simulink model "PBVS_SoftHand"  (R2020b)
settings: Solver=VariableStepAuto  StartTime=0.0  StopTime=10  RelTol=1e-3
model workspace (MAT data in the model file):
  SL_ROS_VariableLengthArrays_MaxSizes.CommonInfo.ArrayTruncateAction = 'EmitWarning'
  SL_ROS_VariableLengthArrays_MaxSizes.MsgTypeMap = containers.Map
  SL_ROS_VariableLengthArrays_MaxSizes.MsgTypeMap.serialization.keys = {'sensor_msgs/Image'}
  SL_ROS_VariableLengthArrays_MaxSizes.MsgTypeMap.serialization.values{1}(1).PropertyName = 'Data'
  SL_ROS_VariableLengthArrays_MaxSizes.MsgTypeMap.serialization.values{1}(1).DataType = 'uint8'
  SL_ROS_VariableLengthArrays_MaxSizes.MsgTypeMap.serialization.values{1}(1).MaxLength = 2800000
  SL_ROS_VariableLengthArrays_MaxSizes.MsgTypeMap.serialization.values{1}(2).PropertyName = 'Encoding'
  SL_ROS_VariableLengthArrays_MaxSizes.MsgTypeMap.serialization.values{1}(2).DataType = 'uint8'
  SL_ROS_VariableLengthArrays_MaxSizes.MsgTypeMap.serialization.values{1}(2).MaxLength = 128
  SL_ROS_VariableLengthArrays_MaxSizes.MsgTypeMap.serialization.uniformity = 0
  SL_ROS_VariableLengthArrays_MaxSizes.MsgTypeMap.serialization.keyType = 'char'
  SL_ROS_VariableLengthArrays_MaxSizes.MsgTypeMap.serialization.valueType = 'any'
values from neighbouring files (symbols this model uses):
  camera_offset = rot(pi, 0, 0) * [-0.10; 0.0; -0.10]    [init_PBVS_SoftHand.m]
  dT = 1/frequency    (= 0.01)    [init_PBVS_SoftHand.m]
  DT = 1/20    (= 0.05)    [init_PBVS_SoftHand.m]
  f = 0.0019    [init_PBVS_SoftHand.m]
  init_pose = [position(1:3); orientation']    [init_PBVS_SoftHand.m]
  Kd = 0.*eye(6)    [init_PBVS_SoftHand.m]
  Kh = eye(7)    [init_PBVS_SoftHand.m]
  Kp = 1.0*eye(6)    [init_PBVS_SoftHand.m]
  l1 = 0.06    [init_PBVS_SoftHand.m]
  l2 = 0.04    [init_PBVS_SoftHand.m]
  O = [0; 0; 0]    [init_PBVS_SoftHand.m]
  o = [0; 0; pi/2-pi/8]    [init_PBVS_SoftHand.m]
  p = [0.5; 0.4; 0.1]    [init_PBVS_SoftHand.m]
  P0 = eye(6)*1    [init_PBVS_SoftHand.m]
  plane_x = 0.008    [init_PBVS_SoftHand.m]
  plane_y = 0.004    [init_PBVS_SoftHand.m]
  Q = zeros(6)    [init_PBVS_SoftHand.m]
  q_init = [ (0.0) (-pi/8) (0.0) (-pi/2-pi/6) (0.0) (pi/2+pi/24) (0.0) ]    [init_PBVS_SoftHand.m]
  R = eye(6)*0.0001    [init_PBVS_SoftHand.m]
  R_cam = rot(phi, theta, psi)    [init_PBVS_SoftHand.m]
  ref = [0; 0; 0.1; 0;  0; -pi]    [init_PBVS_SoftHand.m]
  st = 0.05    [init_PBVS_SoftHand.m]
libraries: simulink x2, robotmaniplib x2
settings Model: Creator=Acer  LastModifiedBy=Acer
settings OptimizationCC: EnhancedBackFolding=on  PassReuseOutputArgsAs=Individual arguments  ZeroExternalMemoryAtStartup=off  ZeroInternalMemoryAtStartup=off  MaxStackSize=64  OptimizeBlockOrder=speed  DifferentSizesBufferReuse=on  OptimizationCustomize=off  EfficientTunableParamExpr=on
settings DebuggingCC: ParameterTunabilityLossMsg=error
settings HardwareCC: ProdBitPerPointer=32  ProdBitPerSizeT=32  ProdBitPerPtrDiffT=32  ProdLargestAtomicFloat=None  ProdIntDivRoundTo=Undefined  ProdEndianess=Unspecified  ProdWordSize=32  ProdHWDeviceType=Generic->Unspecified (assume 32-bit Generic)  UseEmbeddedCoderFeatures=off
settings SFSimCC: MATLABDynamicMemAlloc=off
settings RTWCC: Description=Embedded Coder  SystemTargetFile=ert.tlc  HardwareBoard=Robot Operating System (ROS)  TLCOptions="-aInlineSetEventsForThisBaseRateFcn=TLC_FALSE -aSuppressMultiTaskScheduler=TLC_FALSE  -aRateBasedStepFcn=0"  TemplateMakefile=ert_default_tmf  Toolchain=Catkin  TargetLang=C++
settings CodeAppCC: ForceParamTrailComments=on  IgnoreCustomStorageClasses=off  OperatorAnnotations=on  SimulinkDataObjDesc=on  SFDataObjDesc=on  InsertBlockDesc=on
settings ERTTargetCC: SupportNonInlinedSFcns=on

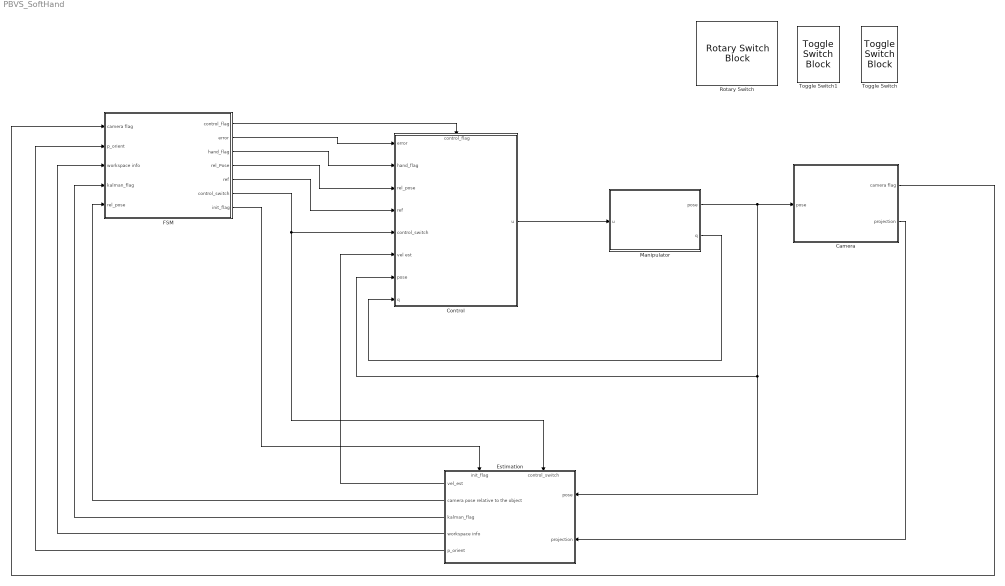
== system PBVS_SoftHand ==
  Camera : Subsystem
  Control : Subsystem
      settings: PortSchema="{\"entries\":[{\"content\":{\"sides\":[{\"content\":{\"connectorIds\":[\"In1\",\"In2\",\"In3\",\"In4\",\"In5\",\"In6\",\"In7\",\"In8\"]},\"type\":\"ConnectorPlacement.EquallySpacedRectSide\",\"uuid\":\"af17fae2-36f6-4efd-b4ba-fb8d1f73429e\"},{\"content\":{\"connectorIds\":[\"Out1\"],\"side\":\"RIGHT\"},\"type\":\"ConnectorPlacement.EquallySpacedRectSide\",\"uuid\":\"2b8fdab6-bdef-4319-b746-176742d42689\"},{\"content\":{\"connectorIds\":[\"In9\"],\"side\":\"TOP\"},\"type\":\"ConnectorPlacement.EquallySpacedRectSide\",\"uuid\":\"e47b4a6a-66e6-45a0-98f9-e5ee84c20568\"},{\"content\":{\"connectorIds\":[],\"side\":\"HIDDEN\"},\"type\":\"ConnectorPlacement.EquallySpacedRectSide\",\"uuid\":\"9d3dc715-f15e-4844-9864-7097570c16fc\"}]},\"type\":\"ConnectorPlacement.EquallySpacedConnector\",\"uuid\":\"752007b5-316d-48d1-9942-1c7a203faf23\"}],\"packageUris\":[\"http://schema.mathworks.com/mf0/Connector/R2020b\"],\"version\":\"1.0\"}"
  Estimation : Subsystem
      settings: PortSchema="{\"entries\":[{\"content\":{\"sides\":[{\"content\":{\"connectorIds\":[\"In1\",\"In2\"]},\"type\":\"ConnectorPlacement.EquallySpacedRectSide\",\"uuid\":\"a08c32dc-abe6-4f2b-ae77-c4d2f876d1ca\"},{\"content\":{\"connectorIds\":[\"Out1\",\"Out2\",\"Out3\",\"Out4\",\"Out5\"],\"side\":\"RIGHT\"},\"type\":\"ConnectorPlacement.EquallySpacedRectSide\",\"uuid\":\"a9594212-1ad7-4004-b7e9-4ae8430051bc\"},{\"content\":{\"connectorIds\":[\"In3\",\"In4\"],\"side\":\"TOP\"},\"type\":\"ConnectorPlacement.EquallySpacedRectSide\",\"uuid\":\"c64d48d0-945a-48a3-9b1a-7425a2bac4f1\"},{\"content\":{\"connectorIds\":[],\"side\":\"HIDDEN\"},\"type\":\"ConnectorPlacement.EquallySpacedRectSide\",\"uuid\":\"141999d7-d8a1-4566-a0df-60055f832239\"}]},\"type\":\"ConnectorPlacement.EquallySpacedConnector\",\"uuid\":\"574f16a2-9616-413e-b861-7d1dd0d71272\"}],\"packageUris\":[\"http://schema.mathworks.com/mf0/Connector/R2020b\"],\"version\":\"1.0\"}"
  FSM : Subsystem
  Manipulator : Subsystem
  Rotary Switch : RotarySwitchBlock  LabelPosition=Bottom
      settings: Values={{'Off', 'Low', 'Medium', 'High'}, [0 -0.02 -0.04 -0.06]}
  Toggle Switch : ToggleSwitchBlock  LabelPosition=Bottom
      settings: Values={{'Off', 'On'}, [0 1]}
  Toggle Switch1 : ToggleSwitchBlock  LabelPosition=Bottom
      settings: Values={{'Off', 'On'}, [0 1]}
  wires:
  Control/1(u) -> Manipulator/1(u)
  Manipulator/1(pose) -> Camera/1(pose), Estimation/1(pose), Control/7(pose)
  Estimation/2(camera pose relative to the object) -> FSM/5(rel_pose)
  Estimation/1(vel_est) -> Control/6(vel est)
  FSM/2(error) -> Control/1(error)
  Estimation/3(kalman_flag) -> FSM/4(kalman_flag)
  FSM/1(control_flag) -> Control/9(control_flag)
  FSM/7(init_flag) -> Estimation/4(init_flag)
  Camera/1(camera flag) -> FSM/1(camera flag)
  FSM/3(hand_flag) -> Control/2(hand_flag)
  Camera/2(projection) -> Estimation/2(projection)
  Estimation/4(workspace info) -> FSM/3(workspace info)
  FSM/4(rel_Pose) -> Control/3(rel_pose)
  Manipulator/2(q) -> Control/8(q)
  Estimation/5(p_orient) -> FSM/2(p_orient)
  FSM/5(ref) -> Control/4(ref)
  FSM/6(control_switch) -> Estimation/3(control_switch), Control/5(control_switch)

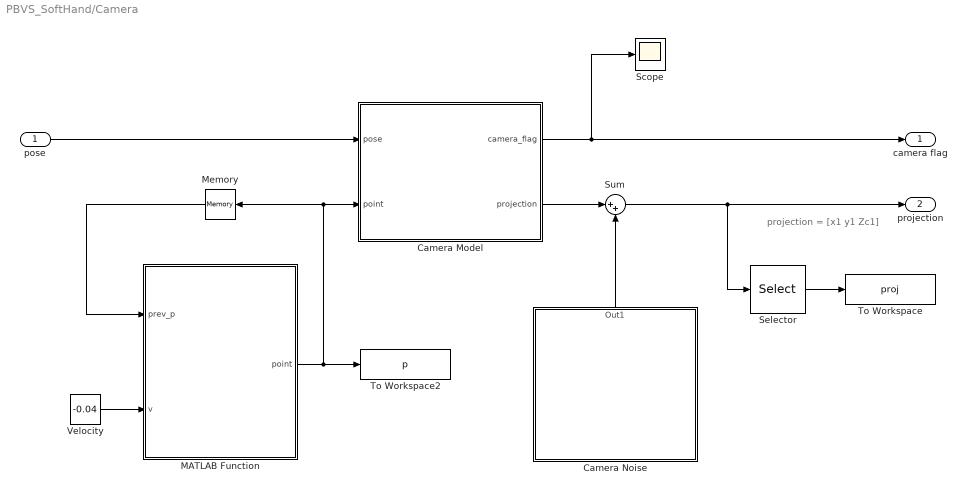
== system PBVS_SoftHand/Camera ==
  note: projection = [x1 y1 Zc1]
  pose : Inport
  Camera Model : MATLAB Function  TreatAsAtomicUnit=on
  Camera Noise : Subsystem
  MATLAB Function : MATLAB Function  TreatAsAtomicUnit=on  SystemSampleTime=dT
  Memory : Memory  InitialCondition=[p; o]
  Scope : Scope
  Selector : Selector  InputPortWidth=12  IndexOptions=Index vector (dialog)  Indices=[1 2 4 5 7 8 10 11]  OutputSizes=1
  Sum : Sum  Inputs=|++
  To Workspace : ToWorkspace  VariableName=proj  SampleTime=st
  To Workspace2 : ToWorkspace  VariableName=p  SampleTime=st
  Velocity : Constant  Value=-0.04  SampleTime=dT
  camera flag : Outport
  projection : Outport  Port=2
  wires:
  pose/1 -> Camera Model/1(pose)
  Selector/1 -> To Workspace/1
  Camera Model/2(projection) -> Sum/1
  Sum/1 -> Selector/1, projection/1
  MATLAB Function/1(point) -> To Workspace2/1, Memory/1, Camera Model/2(point)
  Memory/1 -> MATLAB Function/1(prev_p)
  Velocity/1 -> MATLAB Function/2(v)
  Camera Model/1(camera_flag) -> Scope/1, camera flag/1
  Camera Noise/1(Out1) -> Sum/2

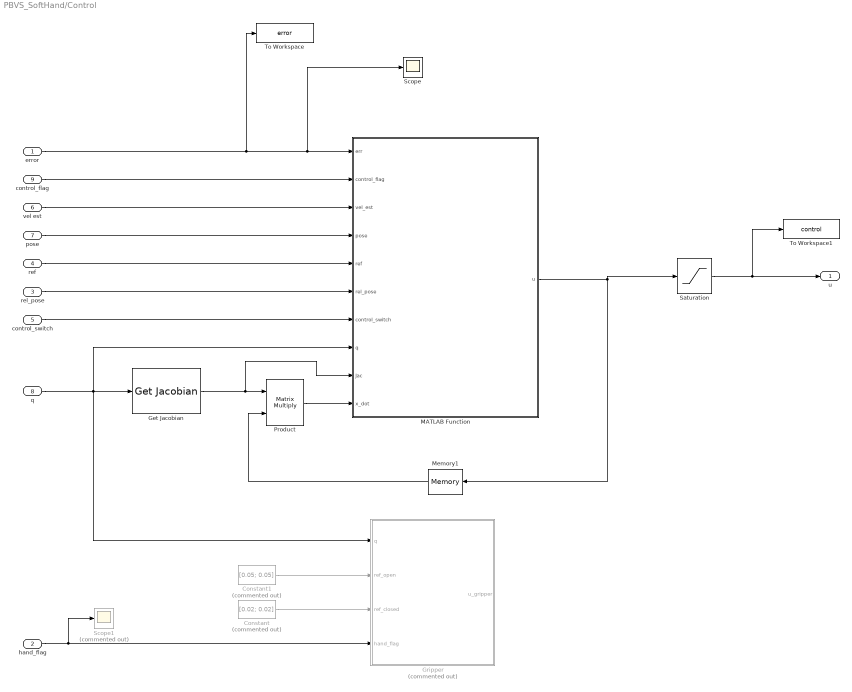
== system PBVS_SoftHand/Control ==
  error : Inport
  hand_flag : Inport  Port=2
  rel_pose : Inport  Port=3
  ref : Inport  Port=4
  control_switch : Inport  Port=5
  vel est : Inport  Port=6
  pose : Inport  Port=7
  q : Inport  Port=8
  control_flag : Inport  Port=9
  Constant : Constant  Commented=on  Value=[0.02; 0.02]
  Constant1 : Constant  Commented=on  Value=[0.05; 0.05]
  Get Jacobian : robotmaniplib/Get Jacobian  RigidBodyTree=robot  EndEffector=right_hand  SimulateUsing=Interpreted execution
      settings: SourceProductBaseCode=RO
  Gripper : MATLAB Function  Commented=on  TreatAsAtomicUnit=on  SystemSampleTime=dT
  MATLAB Function : MATLAB Function  TreatAsAtomicUnit=on  SystemSampleTime=dT
  Memory1 : Memory  InitialCondition=zeros(7,1)
  Product : Product  Multiplication=Matrix(*)
  Saturation : Saturate  UpperLimit=2.5  LowerLimit=-2.5
  Scope : Scope
  Scope1 : Scope  Commented=on
  To Workspace : ToWorkspace  VariableName=error  SampleTime=st
  To Workspace1 : ToWorkspace  VariableName=control  SampleTime=st
  u : Outport
  wires:
  error/1 -> To Workspace/1, Scope/1, MATLAB Function/1(err)
  MATLAB Function/1(u) -> Saturation/1, Memory1/1
  q/1 -> MATLAB Function/8(q), Gripper/1(q), Get Jacobian/1
  Get Jacobian/1 -> MATLAB Function/9(Jac), Product/1
  pose/1 -> MATLAB Function/4(pose)
  Product/1 -> MATLAB Function/10(x_dot)
  Memory1/1 -> Product/2
  vel est/1 -> MATLAB Function/3(vel_est)
  control_flag/1 -> MATLAB Function/2(control_flag)
  hand_flag/1 -> Scope1/1, Gripper/4(hand_flag)
  Constant1/1 -> Gripper/2(ref_open)
  Constant/1 -> Gripper/3(ref_closed)
  Saturation/1 -> To Workspace1/1, u/1
  rel_pose/1 -> MATLAB Function/6(rel_pose)
  ref/1 -> MATLAB Function/5(ref)
  control_switch/1 -> MATLAB Function/7(control_switch)

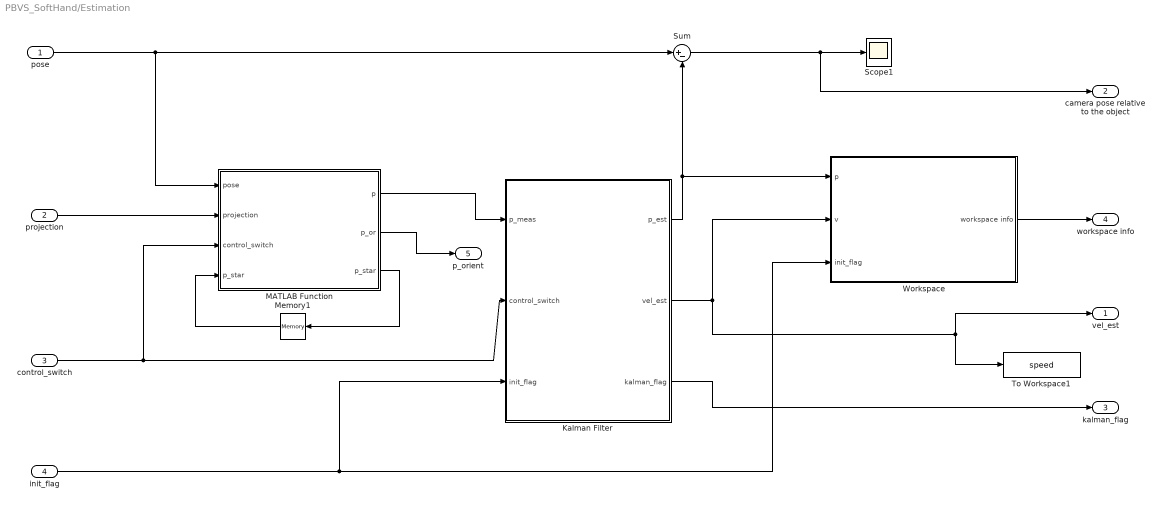
== system PBVS_SoftHand/Estimation ==
  pose : Inport
  projection : Inport  Port=2
  control_switch : Inport  Port=3
  init_flag : Inport  Port=4
  Kalman Filter : Subsystem
  MATLAB Function : MATLAB Function  TreatAsAtomicUnit=on
  Memory1 : Memory  InitialCondition=zeros(6,1)
  Scope1 : Scope
  Sum : Sum  Inputs=|+-
  To Workspace1 : ToWorkspace  VariableName=speed  SampleTime=st
  Workspace : Subsystem
  vel_est : Outport
  camera pose relative to the object : Outport  Port=2
  kalman_flag : Outport  Port=3
  workspace info : Outport  Port=4
  p_orient : Outport  Port=5
  wires:
  projection/1 -> MATLAB Function/2(projection)
  Kalman Filter/2(vel_est) -> vel_est/1, To Workspace1/1, Workspace/2(v)
  pose/1 -> Sum/1, MATLAB Function/1(pose)
  Sum/1 -> Scope1/1, camera pose relative to the object/1
  Kalman Filter/1(p_est) -> Workspace/1(p), Sum/2
  Kalman Filter/3(kalman_flag) -> kalman_flag/1
  init_flag/1 -> Workspace/3(init_flag), Kalman Filter/3(init_flag)
  control_switch/1 -> MATLAB Function/3(control_switch), Kalman Filter/2(control_switch)
  MATLAB Function/3(p_star) -> Memory1/1
  Memory1/1 -> MATLAB Function/4("p_star ")
  Workspace/1(workspace info) -> workspace info/1
  MATLAB Function/1(p) -> Kalman Filter/1(p_meas)
  MATLAB Function/2(p_or) -> p_orient/1

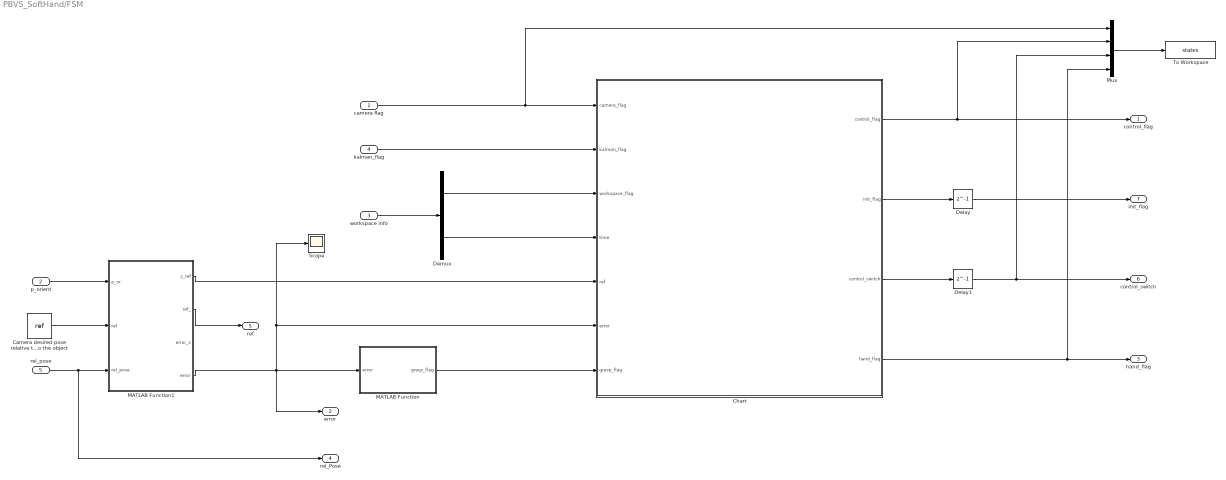
== system PBVS_SoftHand/FSM ==
  camera flag : Inport
  p_orient : Inport  Port=2
  workspace info : Inport  Port=3
  kalman_flag : Inport  Port=4
  rel_pose : Inport  Port=5
  Camera desired pose relative to the object : Constant  Value=ref  SampleTime=-1
  Chart : Stateflow chart  TreatAsAtomicUnit=on
      settings: PortSchema="{\"entries\":[{\"content\":{\"sides\":[{\"content\":{\"connectorIds\":[\"In1\",\"In2\",\"In3\",\"In4\",\"In5\",\"In7\",\"In6\"]},\"type\":\"ConnectorPlacement.EquallySpacedRectSide\",\"uuid\":\"36481a4d-886a-4e43-81c1-a35977eb8c82\"},{\"content\":{\"connectorIds\":[\"Out1\",\"Out2\",\"Out3\",\"Out4\"],\"side\":\"RIGHT\"},\"type\":\"ConnectorPlacement.EquallySpacedRectSide\",\"uuid\":\"35110049-2785-4c15-b5c6-481c07ac5a1c\"},{\"content\":{\"connectorIds\":[],\"side\":\"TOP\"},\"type\":\"ConnectorPlacement.EquallySpacedRectSide\",\"uuid\":\"1a5eb0fb-e0da-4493-abfd-d89cfea2bbc9\"},{\"content\":{\"connectorIds\":[],\"side\":\"HIDDEN\"},\"type\":\"ConnectorPlacement.EquallySpacedRectSide\",\"uuid\":\"1a16b6df-3a60-4de0-94cd-4dad1b3b3a18\"}]},\"type\":\"ConnectorPlacement.EquallySpacedConnector\",\"uuid\":\"816824d5-b448-4026-b485-0d99ee53de77\"}],\"packageUris\":[\"http://schema.mathworks.com/mf0/Connector/R2020b\"],\"version\":\"1.0\"}"
  Delay : Delay  DelayLength=1
  Delay1 : Delay  DelayLength=1
  Demux : Demux  Outputs=2
  MATLAB Function : MATLAB Function  TreatAsAtomicUnit=on
  MATLAB Function1 : MATLAB Function  TreatAsAtomicUnit=on
  Mux : Mux
  Scope : Scope
  To Workspace : ToWorkspace  VariableName=states  SampleTime=st
  control_flag : Outport
  error : Outport  Port=2
  hand_flag : Outport  Port=3
  rel_Pose : Outport  Port=4
  ref : Outport  Port=5
  control_switch : Outport  Port=6
  init_flag : Outport  Port=7
  wires:
  kalman_flag/1 -> Chart/2(kalman_flag)
  Chart/1(control_flag) -> Mux/2, control_flag/1
  camera flag/1 -> Chart/1(camera_flag), Mux/1
  Chart/2(init_flag) -> Delay/1
  Delay/1 -> init_flag/1
  Mux/1 -> To Workspace/1
  Chart/4(hand_flag) -> Mux/4, hand_flag/1
  MATLAB Function/1(grasp_flag) -> Chart/6(grasp_flag)
  workspace info/1 -> Demux/1
  Demux/1 -> Chart/3(workspace_flag)
  Demux/2 -> Chart/4(time)
  Camera desired pose relative to the object/1 -> MATLAB Function1/2(ref)
  p_orient/1 -> MATLAB Function1/1(p_or)
  MATLAB Function1/2(ref_) -> ref/1
  Chart/3(control_switch) -> Delay1/1
  Delay1/1 -> Mux/3, control_switch/1
  MATLAB Function1/1(z_ref) -> Chart/5(ref)
  rel_pose/1 -> rel_Pose/1, MATLAB Function1/3(rel_pose)
  MATLAB Function1/4(error) -> Scope/1, Chart/7(error), error/1, MATLAB Function/1(error)

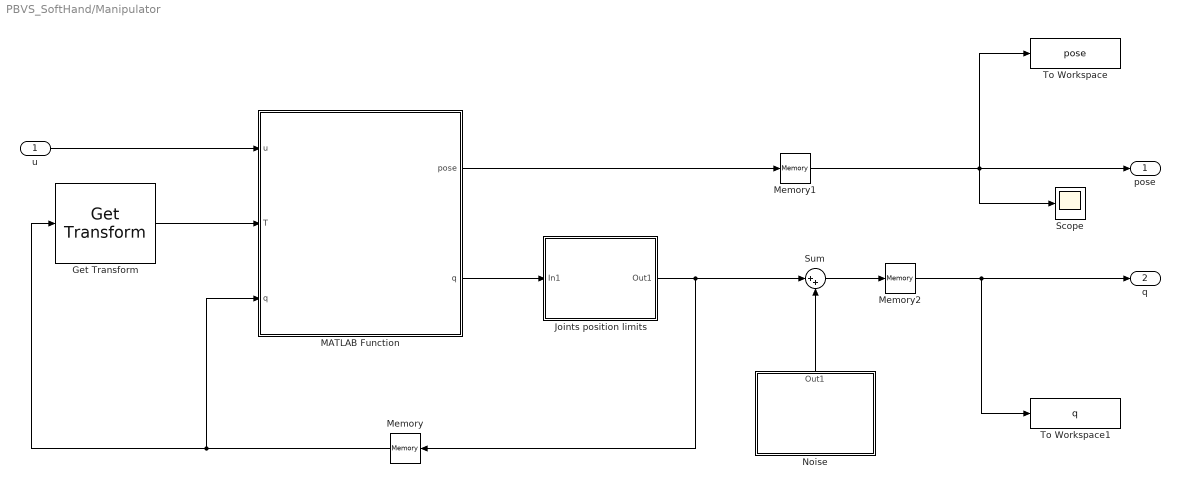
== system PBVS_SoftHand/Manipulator ==
  u : Inport
  Get Transform : robotmaniplib/Get Transform  RigidBodyTree=robot  SourceBody=panda_link0  TargetBody=right_hand  SimulateUsing=Interpreted execution
  Joints position limits : Subsystem
  MATLAB Function : MATLAB Function  TreatAsAtomicUnit=on  SystemSampleTime=dT
  Memory : Memory  InitialCondition=q_init
  Memory1 : Memory  InitialCondition=init_pose
  Memory2 : Memory  InitialCondition=q_init
  Noise : Subsystem
  Scope : Scope
  Sum : Sum  Inputs=|++
  To Workspace : ToWorkspace  VariableName=pose  SampleTime=st
  To Workspace1 : ToWorkspace  VariableName=q  SampleTime=st
  pose : Outport
  q : Outport  Port=2
  wires:
  Memory/1 -> MATLAB Function/3("q "), Get Transform/1
  Get Transform/1 -> MATLAB Function/2(T)
  MATLAB Function/1(pose) -> Memory1/1
  Memory1/1 -> Scope/1, pose/1, To Workspace/1
  u/1 -> MATLAB Function/1(u)
  Sum/1 -> Memory2/1
  Memory2/1 -> q/1, To Workspace1/1
  Joints position limits/1(Out1) -> Sum/1, Memory/1
  MATLAB Function/2(q) -> Joints position limits/1(In1)
  Noise/1(Out1) -> Sum/2

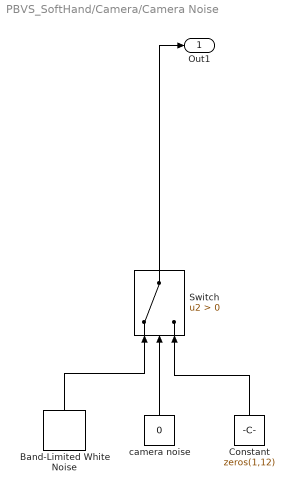
== system PBVS_SoftHand/Camera/Camera Noise ==
  Band-Limited White Noise : simulink/Sources/Band-Limited White Noise  Cov=[0.0000001 0.0000001 0.0000001 0.0000001 0.0000001 0.0000001 0.0000001 0.0000001 0.0000001 0.0000001 0.0000001 0.0000001]  Ts=0.01  seed=[23341 10 14 23341 10 14 23341 10 14 23341 10 14]
  Constant : Constant  Value=zeros(1,12)
  Switch : Switch  Criteria=u2 > Threshold
  camera noise : Constant  Value=0
  Out1 : Outport
  wires:
  Band-Limited White Noise/1 -> Switch/1
  camera noise/1 -> Switch/2
  Switch/1 -> Out1/1
  Constant/1 -> Switch/3

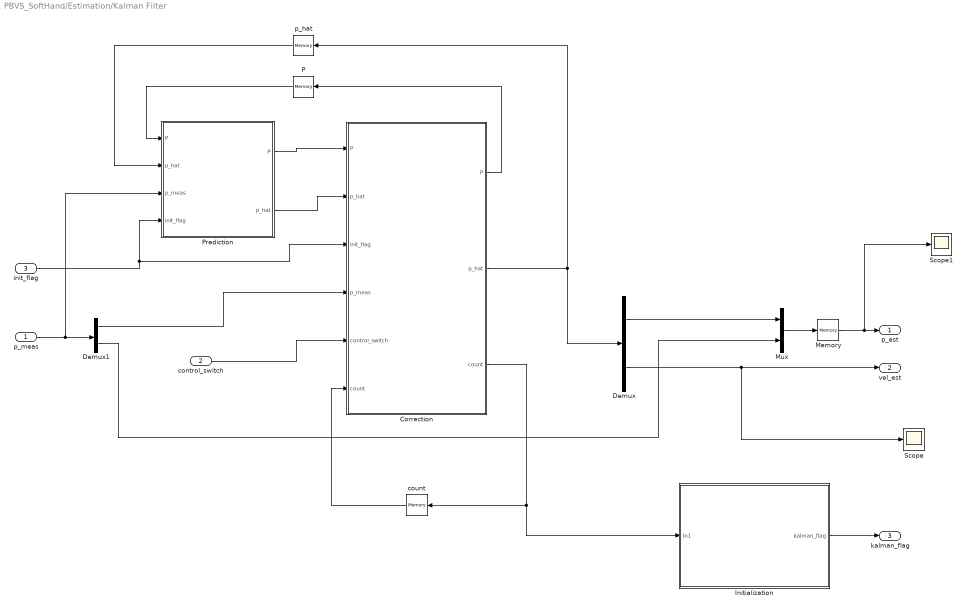
== system PBVS_SoftHand/Estimation/Kalman Filter ==
  p_meas : Inport
  control_switch : Inport  Port=2
  init_flag : Inport  Port=3
  Correction : MATLAB Function  TreatAsAtomicUnit=on  SystemSampleTime=DT
  Demux : Demux  Outputs=2
  Demux1 : Demux  Outputs=2
  Initialization : Subsystem
  Memory : Memory  InitialCondition=zeros(6,1)
  Mux : Mux  Inputs=2
  P : Memory  InitialCondition=P0
  Prediction : MATLAB Function  TreatAsAtomicUnit=on  SystemSampleTime=DT
  Scope : Scope
  Scope1 : Scope
  count : Memory
  p_hat : Memory  InitialCondition=zeros(6,1)
  p_est : Outport
  vel_est : Outport  Port=2
  kalman_flag : Outport  Port=3
  wires:
  Demux/2 -> Scope/1, vel_est/1
  p_hat/1 -> Prediction/2("p_hat ")
  P/1 -> Prediction/1("P ")
  Correction/2(p_hat) -> p_hat/1, Demux/1
  Correction/1(P) -> P/1
  Prediction/1(P) -> Correction/1("P ")
  Prediction/2(p_hat) -> Correction/2("p_hat ")
  p_meas/1 -> Prediction/3(p_meas), Demux1/1
  Mux/1 -> Memory/1
  Demux/1 -> Mux/1
  Demux1/1 -> Correction/4(p_meas)
  Demux1/2 -> Mux/2
  Memory/1 -> Scope1/1, p_est/1
  Correction/3(count) -> Initialization/1(In1), count/1
  count/1 -> Correction/6("count ")
  init_flag/1 -> Prediction/4(init_flag), Correction/3(init_flag)
  Initialization/1(kalman_flag) -> kalman_flag/1
  control_switch/1 -> Correction/5(control_switch)

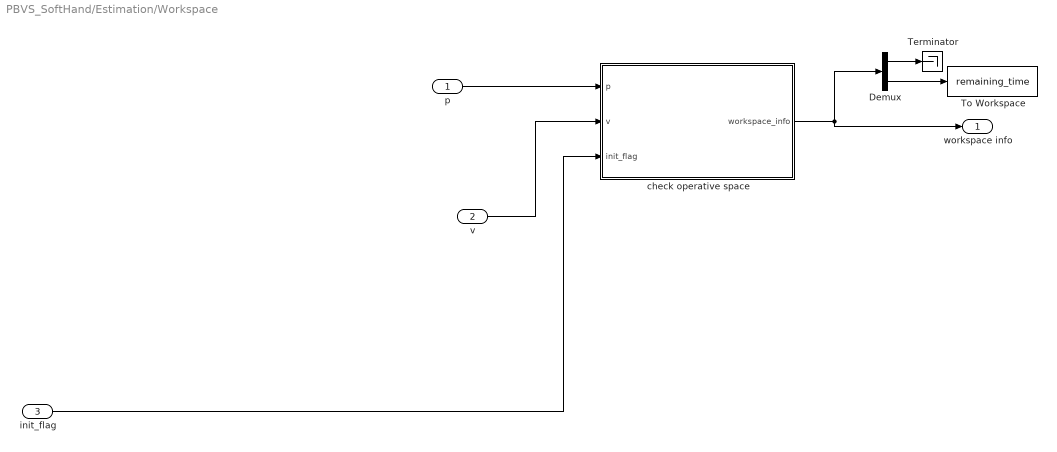
== system PBVS_SoftHand/Estimation/Workspace ==
  p : Inport
  v : Inport  Port=2
  init_flag : Inport  Port=3
  Demux : Demux  Outputs=2
  Terminator : Terminator
  To Workspace : ToWorkspace  VariableName=remaining_time  SampleTime=st
  check operative space : MATLAB Function  TreatAsAtomicUnit=on  SystemSampleTime=1/2
  workspace info : Outport
  wires:
  init_flag/1 -> check operative space/3(init_flag)
  Demux/2 -> To Workspace/1
  Demux/1 -> Terminator/1
  check operative space/1(workspace_info) -> workspace info/1, Demux/1
  p/1 -> check operative space/1(p)
  v/1 -> check operative space/2(v)

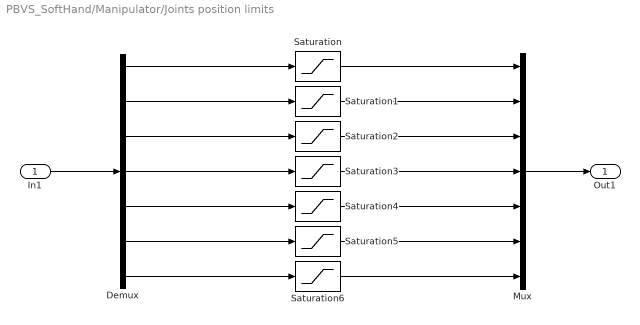
== system PBVS_SoftHand/Manipulator/Joints position limits ==
  In1 : Inport
  Demux : Demux  Outputs=7
  Mux : Mux  Inputs=7
  Saturation{,2,4,6} (4 alike) : Saturate  UpperLimit=166*pi/180  LowerLimit=-166*pi/180
  Saturation1 : Saturate  UpperLimit=101*pi/180  LowerLimit=-101*pi/180
  Saturation3 : Saturate  UpperLimit=-4*pi/180  LowerLimit=-176*pi/180
  Saturation5 : Saturate  UpperLimit=215*pi/180  LowerLimit=-pi/180
  Out1 : Outport
  wires:
  In1/1 -> Demux/1
  Mux/1 -> Out1/1
  Demux/1 -> Saturation/1
  Demux/2 -> Saturation1/1
  Demux/3 -> Saturation2/1
  Demux/4 -> Saturation3/1
  Demux/5 -> Saturation4/1
  Demux/6 -> Saturation5/1
  Demux/7 -> Saturation6/1
  Saturation4/1 -> Mux/5
  Saturation3/1 -> Mux/4
  Saturation2/1 -> Mux/3
  Saturation1/1 -> Mux/2
  Saturation/1 -> Mux/1
  Saturation5/1 -> Mux/6
  Saturation6/1 -> Mux/7

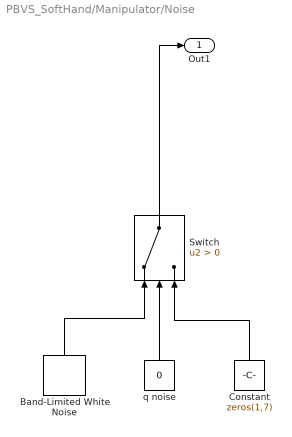
== system PBVS_SoftHand/Manipulator/Noise ==
  Band-Limited White Noise : simulink/Sources/Band-Limited White Noise  Cov=[0.000001 0.000001 0.000001 0.000001 0.000001 0.000001 0.000001]  Ts=0.01  seed=[3341 17 144 12 1 94 2456]
  Constant : Constant  Value=zeros(1,7)
  Switch : Switch  Criteria=u2 > Threshold
  q noise : Constant  Value=0
  Out1 : Outport
  wires:
  Band-Limited White Noise/1 -> Switch/1
  q noise/1 -> Switch/2
  Constant/1 -> Switch/3
  Switch/1 -> Out1/1

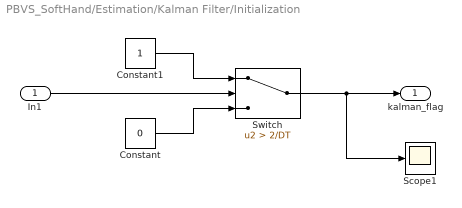
== system PBVS_SoftHand/Estimation/Kalman Filter/Initialization ==
  In1 : Inport
  Constant : Constant  Value=0
  Constant1 : Constant
  Scope1 : Scope
  Switch : Switch  Criteria=u2 > Threshold  Threshold=2/DT
  kalman_flag : Outport
  wires:
  Constant1/1 -> Switch/1
  Constant/1 -> Switch/3
  Switch/1 -> kalman_flag/1, Scope1/1
  In1/1 -> Switch/2

== matlab function PBVS_SoftHand/Estimation/Workspace/check operative space ==
  data: p input; workspace_info output; v input; init_flag input; workspace_dim parameter
function workspace_info = fcn(p, v, init_flag, workspace_dim)

workspace_flag = 0;
remaining_time = 0;
coder.extrinsic('compute_time_ws');

if init_flag == 1
    
    if norm([p(1), p(2)]) < workspace_dim
        
        remaining_time = compute_time_ws(p, v);
        workspace_flag = 1;   
    end
end

workspace_info = [workspace_flag, remaining_time];

== stateflow chart PBVS_SoftHand/FSM/Chart ==
  state Stop
    entry:
    control_flag = 0;
    init_flag = 0;
    hand_flag = 0;
  state ComputeSpeed
    entry:
    control_flag = 0;
    init_flag = 1;
  state TrackTheObject
    entry:
    control_flag = 1;
    control_switch = 0;
  state TrackTheObject_OpenLoop
    entry:
    control_flag = 1;
    control_switch = 1;
  state GraspTheObject
    entry:
    hand_flag = 1;
  (default) -> Stop
  GraspTheObject -> Stop : [workspace_flag == 0]
  TrackTheObject_OpenLoop -> Stop [order 3] : [workspace_flag == 0]
  TrackTheObject -> Stop [order 1] : [camera_flag ==0 || workspace_flag == 0]
  ComputeSpeed -> Stop [order 2] : [camera_flag == 0]
  Stop -> ComputeSpeed : [camera_flag == 1]
  ComputeSpeed -> TrackTheObject [order 1] : [kalman_flag == 1 && workspace_flag == 1 && time > 4]
  TrackTheObject -> TrackTheObject_OpenLoop [order 2] : [abs(error(3))+abs(ref) < 0.25]
  TrackTheObject_OpenLoop -> TrackTheObject [order 2] : [abs(error(3))+abs(ref) > 0.30]
  TrackTheObject_OpenLoop -> GraspTheObject [order 1] : [grasp_flag == 1]
  data: camera_flag input; kalman_flag input; workspace_flag input; time input; ref input; control_flag output; init_flag output; control_switch output; grasp_flag input; hand_flag output; error input

== matlab function PBVS_SoftHand/Control/Gripper ==
  data: q input; ref_open input; ref_closed input; hand_flag input; u_gripper output; Kg parameter
function u_gripper = fcn(q, ref_open, ref_closed, hand_flag, Kg)
% function that computes the gripper control law
% q : joint variables
% ref_open : open gripper desired position 
% ref_closed : closed gripper desired position - used to grasp the object
% hand_flag : flag used to know when the robot can grasp the object
% Kg : gripper gain matrix

u_gripper = zeros(9,1);  % u_gripper initialization

if hand_flag == 1     % gripper close to the object
    
    err_gripper = ref_closed -[q(8); q(9)];
    u_gripper = Kg*[zeros(7,1); err_gripper];   % gripper control law to grasp the object
    
else                  % gripper not close to the object
    err_gripper = ref_open -[q(8); q(9)];
    u_gripper = Kg*[zeros(7,1); err_gripper];   % open gripper control law
    
    
end

== matlab function PBVS_SoftHand/FSM/MATLAB Function1 ==
  data: z_ref output; ref_ output; error_z output; error output; p_or input; ref input; rel_pose input
function [z_ref, ref_, error_z, error] = fcn(p_or, ref, rel_pose)



ref_ = ref;
ref_(4) = (pi/2) * -sign(p_or);
z_ref = ref_(3);


error = zeros(6,1);
error(1:3) = ref_(1:3) - rel_pose(1:3);

R_des = eul2rotm(ref_(4:6)','XYZ');
R_e = eul2rotm(rel_pose(4:6)','XYZ');

quat = rotm2quat(R_des*R_e');

error(4:6) = quat(2:4)';
error_z = error(3);

== matlab function PBVS_SoftHand/Estimation/Kalman Filter/Correction ==
  data: P input; P output; p_hat input; init_flag input; p_hat output; p_meas input; control_switch input; count input; R parameter; count output; P0 parameter
function [P, p_hat, count] = correction(P, p_hat, init_flag, p_meas, control_switch, count, R, P0)
% R : measurement error covariance matrix
% count : counter that increases its value by one at each iteration.
%         When the fortieth iteration is reached, the object velocity is estimated 
%         and the kalman_flag is set to one

if init_flag == 1 && control_switch == 0
    
    C = [eye(3) zeros(3); zeros(3) zeros(3)];
    z = [p_meas; zeros(3,1)];
    
    K = P * C' * (C * P * C' + R)^-1;
    p_hat = p_hat + K * (z - C * p_hat);
    P = (eye(6) - K * C) * P;
    
    count = count + 1;
    
elseif control_switch == 1
    p_hat = p_hat;
    
else
    count = 0;
    P = P0;
    p_hat = zeros(6,1);
end

== matlab function PBVS_SoftHand/Estimation/Kalman Filter/Prediction ==
  data: P input; P output; p_hat input; p_meas input; Q parameter; DT parameter; init_flag input; p_hat output
function [P, p_hat] = prediction(P, p_hat, p_meas, Q, DT, init_flag)
% function that computes the prediction step in Kalman filter
% p_hat : estimated pose of the object
% p_meas : measured pose of the object
% P : estimation error covariance matrix 
% Q : process error covariance matrix
% init_flag : flag used to start Kalman estimation


if p_hat == zeros(6,1)
    p_hat = p_meas;
end

if init_flag == 1
    A = [eye(3) DT*eye(3); zeros(3) eye(3)];
    
    p_hat = A * p_hat;
    P = A * P * A' + Q;
end

== matlab function PBVS_SoftHand/FSM/MATLAB Function ==
  data: error input; grasp_flag output; tolerance parameter
function grasp_flag = fcn(error, tolerance)

grasp_flag = 1;

for i = 1 : length(error)
    
    if abs(error(i)) > tolerance(i)
        grasp_flag = 0;
    end
end

== matlab function PBVS_SoftHand/Control/MATLAB Function ==
  data: err input; control_flag input; vel_est input; Kp parameter; pose input; ref input; rel_pose input; control_switch input; q input; Jac input; u output; x_dot input; Kd parameter; Kh parameter; q_init parameter
function u = fcn(err, control_flag, vel_est, Kp, pose, ref, rel_pose, control_switch, q, Jac, x_dot, Kd, Kh, q_init)

% rel_pose : relative pose between camera and object
% ref : desired relative pose between camera and object
% err : error between desired and actual pose of the camera relative to the object
% vel_est : object estimated velocity from Kalman filter. Used in the
%           control law to reach the moving object.
u = zeros(7, 1);

if (control_flag == 1)

    J = zeros(6, 7);
    ang = rel_pose(4:6) - ref(4:6);
    
    
    %% Trasformation

    Ta = [0     -sin(pose(4))       cos(pose(4))*sin(pose(5)) ;
          0      cos(pose(4))       sin(pose(4))*sin(pose(5)) ;
          1          0                    cos(pose(5))       ];

    if (det(Ta) == 0)
        Ta = eye(3);  
    end

    Rx = [1     0            0      ;
          0 cos(ang(1)) -sin(ang(1));
          0 sin(ang(1)) cos(ang(1))];
    
    Ry = [cos(ang(2)) 0 sin(ang(2)) ;
              0       1     0 ;
         -sin(ang(2)) 0 cos(ang(2))];
    
    Rz = [cos(ang(3)) -sin(ang(3)) 0 ;
          sin(ang(3))  cos(ang(3)) 0 ;
              0            0       1];
    
    Rd = Rz * Ry * Rx;
    
    %% Jacobian
    %J = eye(6);  % Jacobian J(q)
    J(1:3, :) = Jac(4:6, :);
    J(4:6, :) = Jac(1:3, :);
    %
    Ja = [Rd'*eye(3) zeros(3); zeros(3) Rd'*Ta^-1] * J;
    
    J1 = Ja(4:6, :);      % orientation jacobian
    J2 = Ja(1:3, :);      % position jacobian
    pinv_J1 = pinv(J1);
    
    u_vel = [vel_est ; zeros(3,1)]; % control correction to take into account the object velocity
    
    %% PBVS control Law
    if control_switch == 0
        % Closed Loop: Stack of Tasks
        u1 = eye(7)*pinv_J1 * diag([0.7, 1.6, 1.6])* err(4:6);
        P1 = eye(7) - pinv_J1*J1;
        
        u = u1 + pinv(J2*P1)*(J2*u1 + diag([0.7 0.7 0.7/(1+norm(err))])*err(1:3)) + pinv(Ja)*(Kd*x_dot + u_vel); %+ pinv(Ja)*u_vel;
        
    else
        % Open Loop: Classic IBVS Control Law
        u = pinv(Ja) * (Kp * err - Kd * x_dot + u_vel); %+ (eye(7) - pinv(Ja)*Ja) * q0';   %  x_dot = J(q) * q_dot
    end
else
    
    err_init = q_init(1:7)' - q(1:7);
    u = Kh * err_init;
end

== matlab function PBVS_SoftHand/Camera/Camera Model ==
  data: camera_flag output; projection output; f parameter; O parameter; pose input; point input; plane_y parameter; plane_x parameter; l1 parameter; l2 parameter; R_cam parameter; camera_offset parameter
function [camera_flag, projection]= proj(f, O, pose, point, plane_y, plane_x, l1, l2, R_cam, camera_offset)
% function that computes the projection of the point in the image plane
% f : focal lenght
% O : world origin frame
% pose: pose of the camera
% point : object barycentre pose

p = point(1:3);
o = point(4:6);
camera_flag = 0;
d = pose(1:3) - O;    % ee position in world frame
ang = pose(4:6);      % ee orientation      
ang(1) = pose(6);
ang(3) = pose(4);
%%
Rx = [1     0            0       ;
      0 cos(ang(1)) -sin(ang(1)) ;
      0 sin(ang(1))  cos(ang(1))];

Ry = [cos(ang(2)) 0 sin(ang(2)) ;
          0       1     0       ;
     -sin(ang(2)) 0 cos(ang(2))];
 
Rz = [cos(ang(3)) -sin(ang(3)) 0 ;
      sin(ang(3))  cos(ang(3)) 0 ;
          0            0       1];


Rc = Rz * Ry * Rx;

Twe =  [Rc             d;
        zeros(1,3)     1];
  
Tec = [R_cam        camera_offset;          % transformation from camera to end effector
       zeros(1,3)       1];  


%% object points computation

p_1 = p + [-l1/2; -l2/2; 0];
p_2 = p + [-l1/2; +l2/2; 0];
p_3 = p + [l1/2; l2/2; 0];
p_4 = p + [l1/2; -l2/2; 0];

Robj = [cos(o(3)) -sin(o(3)) 0;
        sin(o(3)) cos(o(3))  0;
           0          0      1];
       
p1 = p + Robj * (p_1 - p);
p2 = p + Robj * (p_2 - p);
p3 = p + Robj * (p_3 - p);
p4 = p + Robj * (p_4 - p);

%% 
% POINT 1
P = diag([f,f,1]) * [eye(3), zeros(3,1)]; % camera projection matrix

p_cam1 = Tec^-1 * Twe^-1 * [p1; 1];   % point position in camera frame

p_tilde1 = P * p_cam1;

x_proj1 = p_tilde1(1)/p_cam1(3);
y_proj1 = p_tilde1(2)/p_cam1(3);
Zc1 = p_cam1(3);

projection1  = [x_proj1; y_proj1; Zc1]; %; x_proj2; y_proj2; Zc2];
% x_proj1, y_proj1 : point projection in image plane
% Zc1 : point depth in camera frame


% POINT 2
p_cam2 =  Tec^-1 * Twe^-1 * [p2; 1];   % point position in camera frame

p_tilde2 = P * p_cam2;

x_proj2 = p_tilde2(1)/p_cam2(3);
y_proj2 = p_tilde2(2)/p_cam2(3);
Zc2 = p_cam2(3);

projection2  = [x_proj2; y_proj2; Zc2]; 
% x_proj1, y_proj1 : point projection in image plane
% Zc1 : point depth in camera frame


% POINT 3
p_cam3 =  Tec^-1 * Twe^-1 * [p3; 1];   % point position in camera frame

p_tilde3 = P * p_cam3;

x_proj3 = p_tilde3(1)/p_cam3(3);
y_proj3 = p_tilde3(2)/p_cam3(3);
Zc3 = p_cam3(3);

projection3  = [x_proj3; y_proj3; Zc3];
% x_proj1, y_proj1 : point projection in image plane
% Zc1 : point depth in camera frame


% POINT 4
p_cam4 =  Tec^-1 * Twe^-1 * [p4; 1];   % point position in camera frame

p_tilde4 = P * p_cam4;

x_proj4 = p_tilde4(1)/p_cam4(3);
y_proj4 = p_tilde4(2)/p_cam4(3);
Zc4 = p_cam4(3);

projection4  = [x_proj4; y_proj4; Zc4];
% x_proj1, y_proj1 : point projection in image plane
% Zc1 : point depth in camera frame

projection = [ projection1; projection2; projection3; projection4];

j = 1;
for i = 1 : 4
    if abs(projection(j)) > plane_x || abs(projection(j+1)) > plane_y   % check object visibility
        projection(j) = NaN;
        projection(j+1) = NaN;
        projection(j+2) = NaN;
    end
    j = j + 3;
end


if sum(~isnan(projection)) > 9
    camera_flag = 1;
end

end

== matlab function PBVS_SoftHand/Manipulator/MATLAB Function ==
  data: u input; T input; q input; pose output; dT parameter; O parameter; q output
function [pose, q] = fcn(u, T, q, dT, O)

position = zeros(4, 1);
orientation = zeros(3, 1);
coder.extrinsic('tform2eul');

%% 
q = q + u * dT;

%%

position = T^-1 * [O; 1];
orientation = tform2eul(T^-1, 'ZYX');
pose = [position(1:3); orientation];

== matlab function PBVS_SoftHand/Camera/MATLAB Function ==
  data: prev_p input; point output; v input; dT parameter
function point = fcn(prev_p ,v, dT)

point = prev_p;

point = point + [0; v; 0; 0; 0; 0] * dT;

== matlab function PBVS_SoftHand/Estimation/MATLAB Function ==
  data: p output; p_or output; p_star output; pose input; projection input; control_switch input; O parameter; f parameter; R_cam parameter; camera_offset parameter; p_star input
function [p, p_or, p_star]  = fcn(pose, projection, control_switch, O, f, R_cam, camera_offset, p_star)
% function that computes the point position in camera frame from the point
% projection in the image plane 
% pose : pose of the camera 

projection1 = projection(1:3) ; % projection of the first point
x1 = projection1(1); % x projection in the image plane
y1 = projection1(2); % y projection in the image plane
Zc1 = projection1(3); % point depth in camera frame

projection2 = projection(4:6) ; % projection of the first point
x2 = projection2(1); % x projection in the image plane
y2 = projection2(2); % y projection in the image plane
Zc2 = projection2(3); % point depth in camera frame

projection3 = projection(7:9) ; % projection of the first point
x3 = projection3(1); % x projection in the image plane
y3 = projection3(2); % y projection in the image plane
Zc3 = projection3(3); % point depth in camera frame

projection4 = projection(10:12) ; % projection of the first point
x4 = projection4(1); % x projection in the image plane
y4 = projection4(2); % y projection in the image plane
Zc4 = projection4(3); % point depth in camera frame

d = pose(1:3) - O;    % camera's position in world frame
ang = pose(4:6);      % camera's orientation 
points = zeros(12,1);
p = zeros(6,1);
ang(1) = pose(6);
ang(3) = pose(4);
p_or = 0;
%%
Rx = [1     0            0       ;
      0 cos(ang(1)) -sin(ang(1)) ;
      0 sin(ang(1))  cos(ang(1))];

Ry = [cos(ang(2)) 0 sin(ang(2)) ;
          0       1     0       ;
     -sin(ang(2)) 0 cos(ang(2))];
 
Rz = [cos(ang(3)) -sin(ang(3)) 0 ;
      sin(ang(3))  cos(ang(3)) 0 ;
          0            0       1];


Rc = Rz * Ry * Rx;

Twe =   [Rc             d ;
         zeros(1,3)     1];
  
Tec = [R_cam         camera_offset ;          % transformation from camera to end effector
       zeros(1,3)          1      ];  


   %%
   P = diag([f,f,1]) * [eye(3), zeros(3,1)]; % camera projection matrix
   available_points = zeros(1,4);
    
   if control_switch == 0
   % POINT 1
   if  ~isnan(x1)
       p_tilde1 = [x1 * Zc1; y1 * Zc1; Zc1];
       p_cam1 = P(:, 1:3)^-1 * p_tilde1;
       
       p_hom1 = Twe * Tec * [p_cam1; 1];
       p1 = p_hom1(1:3);     % [p1(1) p1(2) p1(3)] : point position in camera frame
       available_points(1) = 1;
       points(1:3) = p1;
   else
       points(1:3) = NaN(3,1);
   end
   
   
   
   % POINT 2
   if ~isnan(x2)
       p_tilde2 = [x2 * Zc2; y2 * Zc2; Zc2];
       p_cam2 = P(:, 1:3)^-1 * p_tilde2;
       
       p_hom2 = Twe * Tec * [p_cam2; 1];
       p2 = p_hom2(1:3);     % [p1(1) p1(2) p1(3)] : point position in camera frame
       available_points(2) = 1;
       points(4:6) = p2;
   else
       points(4:6) = NaN(3,1);
   end
   
   
   
   % POINT 3
   if ~isnan(x3)
       p_tilde3 = [x3 * Zc3; y3 * Zc3; Zc3];
       p_cam3 = P(:, 1:3)^-1 * p_tilde3;
       
       p_hom3 = Twe * Tec * [p_cam3; 1];
       p3 = p_hom3(1:3);     % [p1(1) p1(2) p1(3)] : point position in camera frame
       available_points(3) = 1;
       points(7:9) = p3;
   else
       points(7:9) = NaN(3,1);
   end
   
   
   
   % POINT 4
   if ~isnan(x4)
       p_tilde4 = [x4 * Zc4; y4 * Zc4; Zc4];
       p_cam4 = P(:, 1:3)^-1 * p_tilde4;
       p_hom4 = Twe * Tec * [p_cam4; 1];
       p4 = p_hom4(1:3);     % [p1(1) p1(2) p1(3)] : point position in camera frame
       available_points(4) = 1;
       points(10:12) = p4;
   else
       points(10:12) = NaN(3,1);
   end
   
   
   switch sum(available_points)
       case 1
           temp_points = zeros(3,1);
           j = 1;
           for i=1:length(points)
               if ~isnan(points(i))
                   temp_points(j) = points(i);
                   j = j + 1;
               end
           end
           p = [temp_points; 0; 0; 0];
           
       case 2
           temp_points = zeros(6,1);
           j = 1;
           for i=1:length(points)
               if ~isnan(points(i))
                   temp_points(j) = points(i);
                   j = j + 1;
               end
           end
           p1 = temp_points(1:3);
           p2 = temp_points(4:6);
           p = [(p1 + p2)/2; 0; 0; 0];
           
       case 3
           temp_points = zeros(9,1);
           j = 1;
           for i=1:length(points)
               if ~isnan(points(i))
                   temp_points(j) = points(i);
                   j = j + 1;
               end
           end
           p1 = temp_points(1:3);
           p2 = temp_points(4:6);
           p3 = temp_points(7:9);
           p = [(p1+p2+p3)/3; 0; 0; 0];
           
       case 4
           p1 = points(1:3);
           p2 = points(4:6);
           p3 = points(7:9);
           p4 = points(10:12);
           o4 = [0; 0; atan2(p4(2)-p1(2),p4(1)-p1(1))];                  % point orientation in world frame
           orient =   [cos(pi/2) 0 sin(pi/2) ;                           % point orientation from world frame to camera frame
               0     1   0    ;
               -sin(pi/2) 0 cos(pi/2)] * o4;
           p = [(p1+p2+p3+p4)/4; orient];
           p_or = orient(1);
           p_star = p;
   end
   
   else
       p = p_star;
       p_or = p_star(4);
   end


% p1 = Twe * pinv(P) * [x1*Zc1; y1*Zc1; Zc1];
% p2 = Twe * pinv(P) * [x2*Zc2; y2*Zc2; Zc2];
